simulink model "sixDOF"  (R2026a)
settings: Solver=ode4  StopTime=30  FixedStep=0.001
values from neighbouring files (symbols this model uses):
  Cd = cdrag.Dc    [dragcurve.m]    (also in dragcurve.mat = [1.038104 1.038104 1.038104 1.038104 1.038104 1.038104 1.038)
  cg_or = cg_or(1:cutoff_idx)    [openrocketdata.m]    (also in rocketMassProps.mat = [1.246677 1.246275 1.245672 1.244766 1.243402 1.241498 1.239)
  cp_or = cp_or(1:cutoff_idx)    [openrocketdata.m]    (also in rocketMassProps.mat = [1.422105 1.424498 1.427709 1.432664 1.438361 1.443278 1.448)
  CP_shift_table = [0 0.02 0.05 0.09 0.14]    [cpShiftData.mat]
  deployPct_table = [0 25 50 75 100]    [cpShiftData.mat]
  Ixx_or = Ixx_or(1:cutoff_idx)    [openrocketdata.m]    (also in rocketMassProps.mat = [0.041252 0.041245 0.041234 0.041218 0.041194 0.04116 0.0411)
  Iyy_or = Iyy_or(1:cutoff_idx)    [openrocketdata.m]    (also in rocketMassProps.mat = [7.47729 7.471945 7.463917 7.45185 7.433695 7.408377 7.38293)
  mass_or = mass_or(1:cutoff_idx)    [openrocketdata.m]    (also in rocketMassProps.mat = [17.606951 17.596657 17.581217 17.558056 17.523315 17.475074)
  thrust = Motor.Thrust    [thrustcurve.m]    (also in thrustcurve.mat = [0 100 1500 2000 2200 1800 1950 2034 2000 1900 1760 1700 ...)
  time = Motor.Time    [thrustcurve.m]    (also in thrustcurve.mat = [0 0.055 0.092 0.1 0.15 0.2 0.5 1 1.5 2 2.5 2.9 ... (16 elem)
  time_c = cdrag.Time    [dragcurve.m]    (also in dragcurve.mat = [0 0.01 0.02 0.03 0.04 0.05 0.055 0.0625 0.0725 0.0825 0.092)
  time_or = time_or(1:cutoff_idx)    [openrocketdata.m]    (also in rocketMassProps.mat = [0.222509 0.233178 0.249181 0.273186 0.309194 0.359194 0.409)
libraries: simulink x4, sharedTrackingLibrary x1
settings Model: LastModifiedBy=Admin

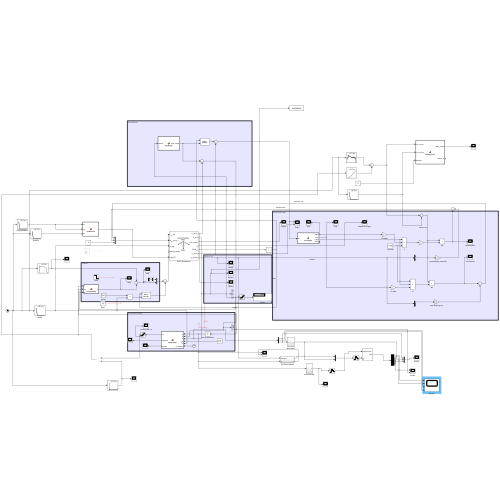
[thumbnail: Simulink's stored preview of the top-level diagram]
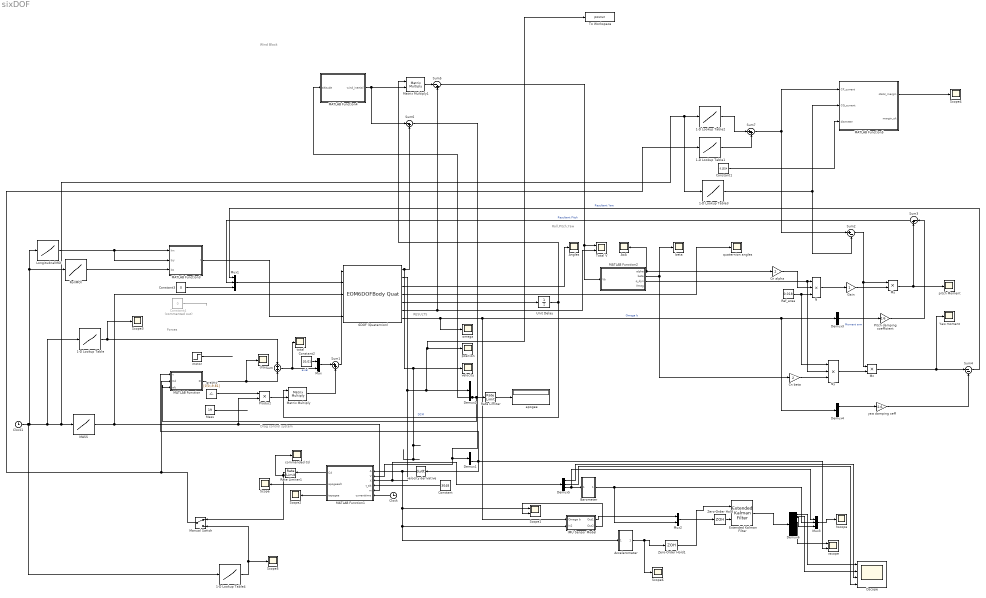
== system sixDOF ==
  note: Wind Block
  note: RESULTS
  note: Roll,Pitch,Yaw
  note: Drag control system
  note: Forces
  1-D Lookup Table : Lookup_n-D  NumberOfTableDimensions=1  BreakpointsForDimension1=time  Table=thrust  ExtrapMethod=Clip  UseLastTableValue=on  InternalRulePriority=Speed  RndMeth=Simplest
  1-D Lookup Table1 : Lookup_n-D  NumberOfTableDimensions=1  BreakpointsForDimension1=deployPct_table  Table=CP_shift_table  InternalRulePriority=Speed  RndMeth=Simplest
  1-D Lookup Table2 : Lookup_n-D  NumberOfTableDimensions=1  BreakpointsForDimension1=time_or  Table=cp_or  ExtrapMethod=Clip  InternalRulePriority=Speed  RndMeth=Simplest
  1-D Lookup Table3 : Lookup_n-D  NumberOfTableDimensions=1  BreakpointsForDimension1=time_or  Table=cg_or  ExtrapMethod=Clip  InternalRulePriority=Speed  RndMeth=Simplest
  1-D Lookup Table4 : Lookup_n-D  NumberOfTableDimensions=1  BreakpointsForDimension1=time_c  Table=Cd  ExtrapMethod=Clip  InternalRulePriority=Speed  RndMeth=Simplest
  6DOF (Quaternion) : EOM6DOFBodyQuat  mtype=Custom Variable  mass_0=19
  Accelerometer : Subsystem
  Angles : Scope
      settings: ActiveDisplayYMinimum=-0.38622595750085542  ActiveDisplayYMaximum=1.7735495845731737  DataLoggingVariableName=ScopeData8
  AoA : Scope
      settings: ActiveDisplayYMinimum=-0.11670515236456694  ActiveDisplayYMaximum=0.1972270518440222  DataLoggingVariableName=ScopeData7
  Barometer : Subsystem
  Clock : Clock
  Clock1 : Clock
  Cn alpha : Gain  Gain=2
  Cn beta : Gain  Gain=2
  Constant : Constant  Value=3048
  Constant1 : Constant  Value=0.1524
  Constant2 : Constant  Value=[0;0]
  Constant3 : Constant  Value=0
  Constant4 : Constant  Commented=on  Value=0
  Demux{1..5} (5 alike) : Demux  Outputs=3
  Demux6 : Demux  Outputs=12
  Dscope : Scope  NumInputPorts=4
      settings: ActiveDisplayYMinimum=-1.2321108597409017E+6  ActiveDisplayYMaximum=1.4308600295046871E+6  DataLoggingVariableName=ScopeData19
  Extended Kalman Filter : sharedTrackingLibrary/Extended Kalman Filter  StateTransitionFcn=StateTransitionFcn  HasStateTransitionJacobianFcn=off  HasAdditiveProcessNoise=Additive  ProcessNoise=Q_matrix  HasTimeVaryingProcessNoise=off  HasStateTransitionFcnExtraArgument=1  InitialState=zeros(12,1)  InitialStateCovariance=eye(12)*0.1  MeasurementFcn1=MeasurementFcn  HasMeasurementJacobianFcn1=off  HasMeasurementEnablePort1=off  HasAdditiveMeasurementNoise1=Additive  MeasurementNoise1=R_matrix  HasTimeVaryingMeasurementNoise1=off  HasMeasurementFcnExtraArgument1=0  HasMeasurementWrapping1=off  HasMeasurementJacobianFcn2=off  HasMeasurementEnablePort2=off  HasAdditiveMeasurementNoise2=Additive  MeasurementNoise2=1  HasTimeVaryingMeasurementNoise2=off  HasMeasurementFcnExtraArgument2=0  HasMeasurementWrapping2=off  HasMeasurementJacobianFcn3=off  HasMeasurementEnablePort3=off  HasAdditiveMeasurementNoise3=Additive  MeasurementNoise3=1  HasTimeVaryingMeasurementNoise3=off  HasMeasurementFcnExtraArgument3=0  HasMeasurementWrapping3=off  HasMeasurementJacobianFcn4=off  HasMeasurementEnablePort4=off  HasAdditiveMeasurementNoise4=Additive  MeasurementNoise4=1  HasTimeVaryingMeasurementNoise4=off  HasMeasurementFcnExtraArgument4=0  HasMeasurementWrapping4=off  HasMeasurementJacobianFcn5=off  HasMeasurementEnablePort5=off  HasAdditiveMeasurementNoise5=Additive  MeasurementNoise5=1  HasTimeVaryingMeasurementNoise5=off  HasMeasurementFcnExtraArgument5=0  HasMeasurementWrapping5=off  EnableMultirate=off  StateTransitionFcnSampleTime=1  MeasurementFcn1SampleTime=1  MeasurementFcn2SampleTime=1  MeasurementFcn3SampleTime=1  MeasurementFcn4SampleTime=1  MeasurementFcn5SampleTime=1  UseCurrentEstimator=on  OutputStateCovariance=off  DataType=double  SampleTime=0.001  NumberOfMeasurements=1
  Gain : Gain
  IMU Sensor Model : Subsystem
  LongitudnalMOI : Lookup_n-D  NumberOfTableDimensions=1  BreakpointsForDimension1=time_or  Table=Iyy_or  ExtrapMethod=Clip  InternalRulePriority=Speed  RndMeth=Simplest
  MASS : Lookup_n-D  NumberOfTableDimensions=1  BreakpointsForDimension1=time_or  Table=mass_or  ExtrapMethod=Clip  InternalRulePriority=Speed  RndMeth=Simplest
  MATLAB Function : MATLAB Function  TreatAsAtomicUnit=on
  MATLAB Function1 : MATLAB Function  TreatAsAtomicUnit=on
  MATLAB Function2 : MATLAB Function  TreatAsAtomicUnit=on
  MATLAB Function3 : MATLAB Function  TreatAsAtomicUnit=on
  MATLAB Function4 : MATLAB Function  TreatAsAtomicUnit=on
  MATLAB Function5 : MATLAB Function  TreatAsAtomicUnit=on
  Manual Switch : ManualSwitch
  Mass : Constant  Value=19
  Matrix Multiply : Product  Multiplication=Matrix(*)
  Matrix Multiply1 : Product  Multiplication=Matrix(*)
  Mux : Mux  Inputs=2
  Mux1 : Mux  Inputs=3
  Mux2 : Mux  Inputs=2
  Mux3 : Mux  Inputs=3
  My : Product
  Mz : Product
  N : Product  Inputs=3
  Ny : Product  Inputs=3
  Pitch damping coefficient : Gain  Gain=2.6
  Product : Product
  Rate Limiter : RateLimiter  RisingSlewLimit=99999  FallingSlewLimit=0  SampleTimeMode=inherited
  Rate Limiter1 : RateLimiter  RisingSlewLimit=2  FallingSlewLimit=-2  SampleTimeMode=inherited
  Ref_area : Constant  Value=0.018
  RollMOI : Lookup_n-D  NumberOfTableDimensions=1  BreakpointsForDimension1=time_or  Table=Ixx_or  ExtrapMethod=Clip  InternalRulePriority=Speed  RndMeth=Simplest
  Scope{,2..6} (6 alike) : Scope
      Scope settings: ActiveDisplayYMinimum=-3975.2759341657311  ActiveDisplayYMaximum=5346.1757277784072  DataLoggingVariableName=ScopeData4
      Scope2 settings: ActiveDisplayYMinimum=23.131664202979607  ActiveDisplayYMaximum=34.456731548921958  DataLoggingVariableName=ScopeData6
      Scope3 settings: ActiveDisplayYMinimum=-765.07484589225214  ActiveDisplayYMaximum=2519.6031220028276  DataLoggingVariableName=ScopeData15
      Scope4 settings: ActiveDisplayYMinimum=1.5294476200072862  ActiveDisplayYMaximum=1.5909519727413044  DataLoggingVariableName=ScopeData20
      Scope5 settings: DataLoggingVariableName=ScopeData21
      Scope6 settings: ActiveDisplayYMinimum=-108.72602500762326  ActiveDisplayYMaximum=165.70364248889467  DataLoggingVariableName=ScopeData22
  Scope1 : Scope  NumInputPorts=2
      settings: ActiveDisplayYMinimum=-195.213202209058  ActiveDisplayYMaximum=201.78596327672926  DataLoggingVariableName=ScopeData16
  Sum : Sum
  Sum1 : Sum  Inputs=|++
  Sum2 : Sum  Inputs=|+-
  Sum3 : Sum  Inputs=|-+
  Sum4 : Sum  Inputs=|--
  Sum5 : Sum  Inputs=|-+
  Sum6 : Sum  Inputs=|-+
  Sum7 : Sum  Inputs=|++
  To Workspace : ToWorkspace  VariableName=posrun  SampleTime=-1
  Total V : Scope  NumInputPorts=2
      settings: ActiveDisplayYMinimum=-119.83899710725643  ActiveDisplayYMaximum=265.49667563260067  DataLoggingVariableName=ScopeData11
  Unit Delay : UnitDelay  SampleTime=-1
  Yaw moment : Scope
      settings: ActiveDisplayYMinimum=-18.650703940874124  ActiveDisplayYMaximum=20.0541694649058  DataLoggingVariableName=ScopeData12
  Zero-Order Hold : ZeroOrderHold  SampleTime=0.001
  Zero-Order Hold1 : ZeroOrderHold  SampleTime=0.001
  apogee : Display
  beta : Scope
      settings: ActiveDisplayYMinimum=-0.79579174295748067  ActiveDisplayYMaximum=0.81085505135714131  DataLoggingVariableName=ScopeData13
  commanded Cd : Scope
      settings: ActiveDisplayYMinimum=0.46813060173680338  ActiveDisplayYMaximum=1.0423365096891759  DataLoggingVariableName=ScopeData5
  drag : Scope
      settings: ActiveDisplayYMinimum=-396.86130675218692  ActiveDisplayYMaximum=62.412916979427223  DataLoggingVariableName=ScopeData2
  gravity : Constant  Value=[0;0;-9.81]  VectorParams1D=off
  hscope : Scope
      settings: ActiveDisplayYMinimum=3011.5000433877526  ActiveDisplayYMaximum=3016.5175693350766  DataLoggingVariableName=ScopeData17
  motor : Step  Time=3.6  InitialValue=1667.8  FinalValue=0  SampleTime=0
  omega : Scope
      settings: ActiveDisplayYMinimum=-1.5223393973231611  ActiveDisplayYMaximum=1.5244987566500803  DataLoggingVariableName=ScopeData9
  pitch Moment : Scope
      settings: ActiveDisplayYMinimum=-72.212026662162884  ActiveDisplayYMaximum=251.70727276885549  DataLoggingVariableName=ScopeData10
  position : Scope
      settings: ActiveDisplayYMinimum=-96.029513978973227  ActiveDisplayYMaximum=1106.717517089746
  quaternion angles : Scope
      settings: ActiveDisplayYMinimum=-1.2402927428054364  ActiveDisplayYMaximum=1.2489214158672706  DataLoggingVariableName=ScopeData14
  total : Scope
      settings: ActiveDisplayYMinimum=-148.90644792235315  ActiveDisplayYMaximum=814.83016826926712  DataLoggingVariableName=ScopeData3
  velocity : Scope
      settings: ActiveDisplayYMinimum=-133.66097006254228  ActiveDisplayYMaximum=352.42758008154624
  velocity derivative : Derivative
  vscope : Scope  NumInputPorts=2
      settings: ActiveDisplayYMinimum=-2316.2800891691668  ActiveDisplayYMaximum=3591.56625908264  DataLoggingVariableName=ScopeData18
  yaw damping ceff : Gain  Gain=2.6
  wires:
  motor/1 -> ?
  MATLAB Function/1(D) -> Sum/2, drag/1
  Sum/1 -> Mux/2, total/1  "axial"
  6DOF (Quaternion)/1 -> velocity/1, Sum6/2
  Demux1/3 -> vscope/2, MATLAB Function/1(v), velocity derivative/1
  velocity derivative/1 -> Scope1/1, Accelerometer/1(In1), IMU Sensor Model/2(In2), MATLAB Function1/1(A)
  Constant/1 -> MATLAB Function1/4(t_alt)
  Clock/1 -> MATLAB Function1/6(currenttime)
  MATLAB Function1/1(Cd) -> Rate Limiter1/1
  Rate Limiter/1 -> apogee/1
  Demux2/3 -> MATLAB Function/3(alt), Rate Limiter/1, MATLAB Function4/1(altitude)
  Manual Switch/1 -> 1-D Lookup Table1/1, MATLAB Function/2(Cd)
  MATLAB Function1/2(apogeealt) -> Scope/1
  MATLAB Function1/3(tapogee) -> Scope2/1
  Sum1/1 -> 6DOF (Quaternion)/1
  gravity/1 -> Product/1
  Mass/1 -> ?
  Product/1 -> Matrix Multiply/2
  6DOF (Quaternion)/5 -> Unit Delay/1
  Unit Delay/1 -> Matrix Multiply1/1, Matrix Multiply/1  "DCM"
  Matrix Multiply/1 -> Sum1/2
  Constant2/1 -> Mux/1
  Mux/1 -> Sum1/1
  Mux1/1 -> 6DOF (Quaternion)/2
  6DOF (Quaternion)/6 -> Total V/2, Sum5/2
  MATLAB Function2/1(alpha) -> Cn alpha/1, AoA/1
  MATLAB Function2/3(q_dyn) -> Ny/2, N/1
  Cn alpha/1 -> N/2
  Ref_area/1 -> N/3, Ny/1
  Sum7/1 -> Sum2/1, MATLAB Function5/1(CP_current)
  1-D Lookup Table3/1 -> Sum2/2, MATLAB Function5/2(CG_current)
  Sum2/1 -> My/1, Mz/1  "Moment arm"
  N/1 -> Gain/1
  Constant4/1 -> ?
  My/1 -> Sum3/2, pitch Moment/1
  6DOF (Quaternion)/3 -> Angles/1
  6DOF (Quaternion)/7 -> Demux3/1, Demux4/1, IMU Sensor Model/1(Omega b), omega/1  "Omega b"
  Gain/1 -> My/2
  Demux3/2 -> Pitch damping coefficient/1
  Pitch damping coefficient/1 -> Sum3/1
  Sum3/1 -> Mux1/2  "Resultant Pitch"
  Ny/1 -> Mz/2
  Mz/1 -> Sum4/1, Yaw moment/1
  MATLAB Function2/2(beta) -> beta/1, Cn beta/1
  Cn beta/1 -> Ny/3
  Constant3/1 -> Mux1/3
  Demux4/1 -> yaw damping ceff/1
  Sum4/1 -> Mux1/1  "Resultant Yaw"
  6DOF (Quaternion)/4 -> quaternion angles/1
  yaw damping ceff/1 -> Sum4/2
  MASS/1 -> Product/2, MATLAB Function1/5(m), 6DOF (Quaternion)/3
  LongitudnalMOI/1 -> MATLAB Function3/2(Iyy), MATLAB Function3/1(Ixx)
  RollMOI/1 -> MATLAB Function3/3(Izz)
  MATLAB Function3/1(I) -> 6DOF (Quaternion)/5
  1-D Lookup Table/1 -> Scope3/1, Sum/1
  IMU Sensor Model/2(Out2) -> Scope1/2
  Demux5/3 -> Mux3/1, Barometer/1(In1)
  Barometer/1(Out1) -> Mux2/2, Mux3/2
  Mux2/1 -> Zero-Order Hold/1
  Zero-Order Hold/1 -> Extended Kalman Filter/2
  Extended Kalman Filter/1 -> Demux6/1
  Demux6/3 -> Mux3/3
  Mux3/1 -> hscope/1
  IMU Sensor Model/1(Out1) -> Mux2/1
  Accelerometer/1(Out1) -> Scope6/1, Zero-Order Hold1/1
  Zero-Order Hold1/1 -> Extended Kalman Filter/1
  MATLAB Function4/1(wind_inertial) -> Sum6/1, Matrix Multiply1/2
  Matrix Multiply1/1 -> Sum5/1
  Sum5/1 -> Total V/1, MATLAB Function2/1(Vb)
  Sum6/1 -> MATLAB Function1/2(V), Demux1/1
  Demux6/6 -> vscope/1
  Demux6/1 -> Dscope/1
  Demux6/2 -> Dscope/2
  Demux5/1 -> Dscope/3
  Demux5/2 -> Dscope/4
  1-D Lookup Table2/1 -> Sum7/1
  1-D Lookup Table1/1 -> Sum7/2
  Constant1/1 -> MATLAB Function5/3(diameter)
  MATLAB Function5/1(static_margin) -> Scope4/1
  6DOF (Quaternion)/2 -> Demux5/1, MATLAB Function1/3(X), To Workspace/1, position/1, Demux2/1
  1-D Lookup Table4/1 -> Scope5/1, Manual Switch/2
  Rate Limiter1/1 -> commanded Cd/1, Manual Switch/1
  Clock1/1 -> 1-D Lookup Table4/1, 1-D Lookup Table3/1, 1-D Lookup Table2/1, MASS/1, 1-D Lookup Table/1, RollMOI/1, LongitudnalMOI/1

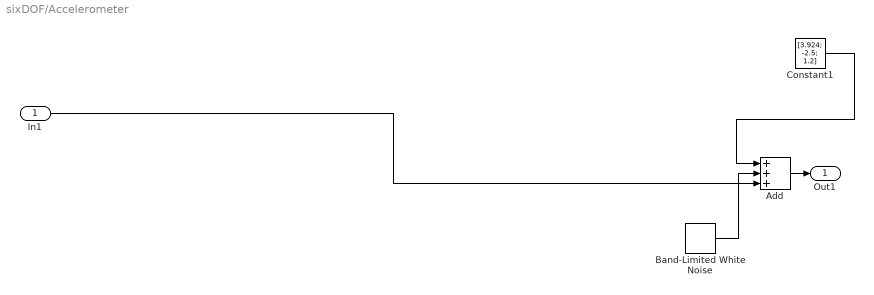
== system sixDOF/Accelerometer ==
  In1 : Inport
  Add : Sum  Inputs=+++
  Band-Limited White Noise : simulink/Sources/Band-Limited White Noise  Cov=[0.00012; 0.00012; 0.00012]  Ts=0.001  seed=[23341]
  Constant1 : Constant  Value=[3.924; -2.5; 1.2]
  Out1 : Outport
  wires:
  Band-Limited White Noise/1 -> Add/2
  Add/1 -> Out1/1
  Constant1/1 -> Add/1
  In1/1 -> Add/3

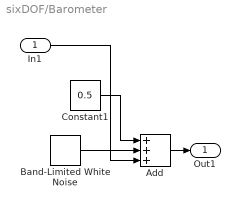
== system sixDOF/Barometer ==
  In1 : Inport
  Add : Sum  Inputs=+++
  Band-Limited White Noise : simulink/Sources/Band-Limited White Noise  Cov=[0.00001]  Ts=0.001  seed=[23341]
  Constant1 : Constant  Value=0.5
  Out1 : Outport
  wires:
  Band-Limited White Noise/1 -> Add/2
  Constant1/1 -> Add/1
  Add/1 -> Out1/1
  In1/1 -> Add/3

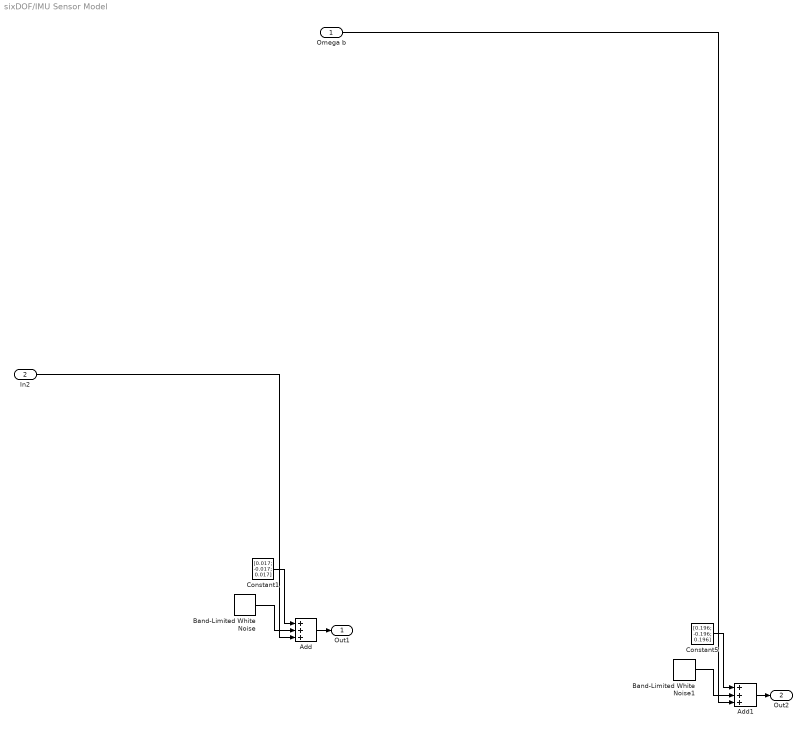
== system sixDOF/IMU Sensor Model ==
  Omega b : Inport
  In2 : Inport  Port=2
  Add : Sum  Inputs=+++
  Add1 : Sum  Inputs=+++
  Band-Limited White Noise : simulink/Sources/Band-Limited White Noise  Cov=[0.0000000000048; 0.0000000000048; 0.0000000000048]  Ts=0.001  seed=[23341]
  Band-Limited White Noise1 : simulink/Sources/Band-Limited White Noise  Cov=[0.00000000047; 0.00000000047; 0.00000000047]  Ts=0.001  seed=[23341]
  Constant1 : Constant  Value=[0.017; -0.017; 0.017]
  Constant5 : Constant  Value=[0.196; -0.196; 0.196]
  Out1 : Outport
  Out2 : Outport  Port=2
  wires:
  In2/1 -> Add/3
  Constant5/1 -> Add1/1
  Band-Limited White Noise/1 -> Add/2
  Band-Limited White Noise1/1 -> Add1/2
  Add1/1 -> Out2/1
  Constant1/1 -> Add/1
  Omega b/1 -> Add1/3
  Add/1 -> Out1/1

== matlab function sixDOF/MATLAB Function1 ==
  data: Cd output; apogeealt output; tapogee output; A input; V input; X input; t_alt input; m input; currenttime input
function [Cd,apogeealt,tapogee] = apogeepred(A,V,X,t_alt,m,currenttime)

apogeeTG = t_alt;

currentAlt= X(3);

currentverticalvel=V(3);

currentverticalacc=A;

persistent alt_lut rho_lut

if isempty(alt_lut)

S = coder.load('atmoData.mat');

alt_lut = S.altitude_data;

rho_lut = S.density_data;

end

Area = 0.018;

Cdclean = 0.3;

vsim = currentverticalvel;

altsim = currentAlt;

t = currenttime;

deltat = 0.01;

apogeealt = 0;

tapogee=0;

if(currentverticalacc > 0)

Cd=Cdclean;

return;

end

for c = 1:18

Cdsim= Cdclean + c*0.03;

for i = 1 : 3000

rho = interp1(alt_lut, rho_lut, altsim, 'linear', 'extrap');

F = -0.5*Cdsim*rho*Area*(vsim^2) - 9.81*m;

asim= F/m;

vsim = vsim + asim*deltat;

altsim = altsim + vsim*deltat;

t=t+deltat;

if(vsim<0)

apogeealt=altsim;

tapogee = t;

break;

end

end

Cd=Cdsim;

if apogeealt < apogeeTG

break;

end

end

== matlab function sixDOF/MATLAB Function ==
  data: v input; D output; Cd input; alt input
function D = ComputeDrag(v,Cd,alt)
A=0.018;
altsim = alt;
persistent alt_lut rho_lut
if isempty(alt_lut)

    S = coder.load('atmoData.mat');

    alt_lut = S.altitude_data;

    rho_lut = S.density_data;

end
rho = interp1(alt_lut, rho_lut, altsim, 'linear', 'extrap');
%Cd=0.3;

D = -0.5*Cd*rho*A*(v^2);
end

== matlab function sixDOF/MATLAB Function2 ==
  data: Vb input; alpha output; beta output; q_dyn output; Vmag output
function [alpha,beta, q_dyn, Vmag] = AeroAngles(Vb)
    u = Vb(1); v = Vb(2); w = Vb(3);
    Vmag = sqrt(u^2 + v^2 + w^2);
    
    if Vmag < 0.1
        alpha = 0;
        beta = 0;
    else
        alpha = atan2(u, w);% pitch-plane angle of attack
        beta = atan2(v,w);
    end
    
    rho = 1.225;   % swap for your lookup table later, same as ComputeDrag
    q_dyn = 0.5*rho*Vmag^2;
end

== matlab function sixDOF/MATLAB Function3 ==
  data: Ixx input; I output; Iyy input; Izz input
function I = buildInertia(Ixx, Iyy, Izz)
    I = diag([Ixx, Iyy, Izz]);
end

== matlab function sixDOF/MATLAB Function4 ==
  data: altitude input; wind_inertial output
function wind_inertial = WindModel(altitude)
    v_ref = 0;      % m/s, reference wind speed
    h_ref = 10;     % m, reference height
    alpha_shear = 0;   % shear exponent, open terrain

    if altitude < 1
        alt_calc = 1;   % avoid singularity near ground
    else
        alt_calc = altitude;
    end

    wind_speed = v_ref * (alt_calc/h_ref)^alpha_shear;

    % Wind direction: assume blowing along inertial X for now
    wind_inertial = [wind_speed; 0; 0];
end

== matlab function sixDOF/MATLAB Function5 ==
  data: CP_current input; static_margin output; CG_current input; diameter input; margin_ok output
function [static_margin, margin_ok] = StabilityCheck(CP_current, CG_current, diameter)
    static_margin = (CP_current - CG_current) / diameter;
    margin_ok = (static_margin >= 1.5) && (static_margin <= 2.5);
end
